simulink model "MSICA_Projet1_StructureControleAugmente"  (R2018a)
settings: Solver=VariableStepAuto  StartTime=0.0  StopTime=10.0  RelTol=1e-3
values from neighbouring files (symbols this model uses):
  A_S1_S2 = [ zeros(3,3) eye(3) ... (first row only)    [DonneesProjet.m]
  B_S1_S2 = [zeros(3,3); inv(M_S1_S2)]    [DonneesProjet.m]
  C1 = [eye(3) zeros(3,3)]    [DonneesProjet.m]
libraries: Blocs_LTI x1
settings Model: Creator=natha  LastModifiedBy=natha
settings DataIOCC: ReturnWorkspaceOutputs=on
settings SFSimCC: SimUseLocalCustomCode=on
settings RTWCC: RTWUseLocalCustomCode=on

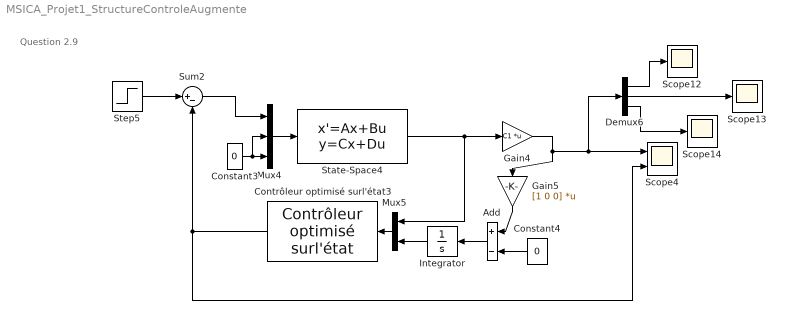
== system MSICA_Projet1_StructureControleAugmente ==
  note: Question 2.9
  Add : Sum  Inputs=+-
  Constant3 : Constant  Value=0
  Constant4 : Constant  Value=0
  Contrôleur optimisé surl'état3 : Blocs_LTI/Contrôleur optimisé surl'état  MaskParameter1=A2  MaskParameter2=B2  MaskParameter3=diag([1e7 1e7 1e7 1e5 1e5 1e5 1e11])  MaskParameter4=eye(1,1)
  Demux6 : Demux  Outputs=3
  Gain4 : Gain  Gain=C1  Multiplication=Matrix(K*u)
  Gain5 : Gain  Gain=[1 0 0]  Multiplication=Matrix(K*u)
  Integrator : Integrator
  Mux4 : Mux  Inputs=3
  Mux5 : Mux  Inputs=2
  Scope12 : Scope
  Scope13 : Scope
  Scope14 : Scope
  Scope4 : Scope  NumInputPorts=2
  State-Space4 : StateSpace  A=A_S1_S2  B=B_S1_S2  C=eye(6)  D=zeros(6,3)  InitialCondition=0
  Step5 : Step  Time=0  After=10  SampleTime=0
  Sum2 : Sum  Inputs=|+-
  wires:
  Constant3/1 -> Mux4/2, Mux4/3
  Mux4/1 -> State-Space4/1
  Step5/1 -> Sum2/1
  Gain5/1 -> Add/1
  Add/1 -> Integrator/1
  Constant4/1 -> Add/2
  Gain4/1 -> Demux6/1, Scope4/1, Gain5/1
  State-Space4/1 -> Mux5/1, Gain4/1
  Demux6/1 -> Scope12/1
  Demux6/3 -> Scope14/1
  Mux5/1 -> Contrôleur optimisé surl'état3/1
  Demux6/2 -> Scope13/1
  Sum2/1 -> Mux4/1
  Integrator/1 -> Mux5/2
  Contrôleur optimisé surl'état3/1 -> Sum2/2, Scope4/2
